simulink model "SimulinkMaster"  (R2025b)
settings: Solver=ode5  StartTime=0.0  StopTime=inf  RelTol=1e-3
undefined symbols (not defined in the file or in its folder): National_Instruments, PCI
libraries: sldrtlib x7, dspstat3 x3
settings Model: Creator=Admin  LastModifiedBy=Admin
settings HardwareCC: ProdBitPerLong=64.0  ProdHWDeviceType=Intel->x86-64 (Linux 64)
settings RTWCC: SystemTargetFile=sldrt.tlc  TemplateMakefile=sldrt.tmf  RTWCompilerOptimization=on  Description=Simulink Desktop Real-Time
settings CodeAppCC: MaxIdLength=95.0
settings SimulinkDesktopRealTimeCC: ExtModeTransport=0.0  ExtModeStaticAllocSize=1000000.0  TargetLibSuffix=_sldrt.a  TargetPreCompLibLocation=C:\Program Files\MATLAB\R2025b\toolbox\sldrt\lib\win64  MultiwordLength=2048.0  DynamicStringBufferSize=256.0  ParMdlRefBuildCompliant=on  PreserveMATLABNamespacesInGeneratedCode=on  SubcomponentCodeInterfacePackaging=Reusable function

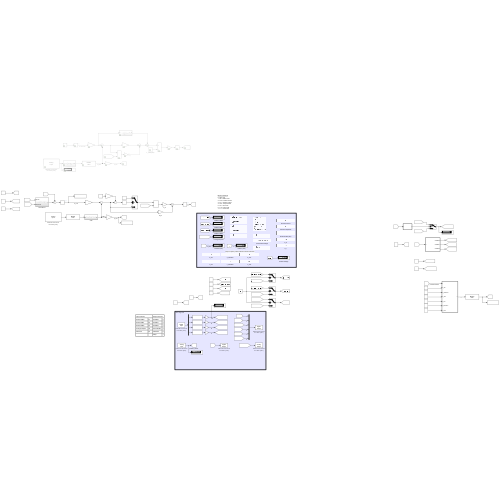
[thumbnail: Simulink's stored preview of the top-level diagram]
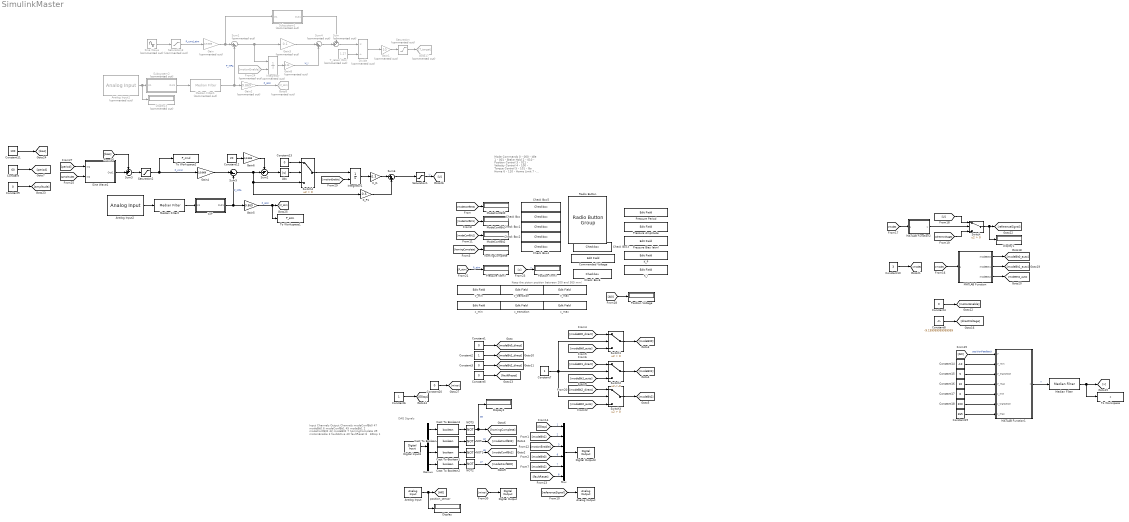
== system SimulinkMaster ==
  note: Keep the piston position between 200 and 365 mm!
  note: Input Channels
      | ​Output Channels
      |
      | modeConfBit0
      | 47
      | modeBit0
      | 6
      |
      | modeConfBit1
      | 45
      | modeBit1
      | 2
      |
      | modeConfBit2
      | 42
      | modeBit2
      | 7
      |
      | homingComplete
      | 39
      | motionEnable
      | 3
      |
      | faultActive
      | 40
      | faultReset
      | 8
      |
      | ​
      | ​
      | EStop
      | 1
  note: DAQ Signals
  note: Mode Commands
      | 0 - 000 - Idle
      | 1 - 001 - Brake Hold
      | 2 - 010 - Position Control
      | 3 - 011 - Velocity Control
      | 4 - 100 - Torque Control
      | 5 - 101 - Go Home
      | 6 - 110 - Home Limit
      | 7 - 111 - Home EOT
  Abs : Abs  SaturateOnIntegerOverflow=off
  Analog Input : sldrtlib/Analog Input  SampleTime=0.003  MaxMissedTicks=1e6  ShowMissedTicks=off  YieldWhenWaiting=off  DrvName=National_Instruments/PCI-6251  DrvAddress=4294967295  DrvOptions=[1 255 0 0 0]  Channels=[1]  RangeMode=1  VoltRange=1  DataType=1
      settings: AttributesFormatString=National Instruments\nPCI-6251 [auto]
  Analog Input1 : sldrtlib/Analog Input  Commented=on  SampleTime=0.003  MaxMissedTicks=1e6  ShowMissedTicks=off  YieldWhenWaiting=off  DrvName=National_Instruments/PCI-6251  DrvAddress=4294967295  DrvOptions=[1 255 0 0 0]  Channels=3  RangeMode=1  VoltRange=1  DataType=1
      settings: AttributesFormatString=National Instruments\nPCI-6251 [auto]
  Analog Input2 : sldrtlib/Analog Input  SampleTime=0.003  MaxMissedTicks=1e6  ShowMissedTicks=off  YieldWhenWaiting=off  DrvName=National_Instruments/PCI-6251  DrvAddress=4294967295  DrvOptions=[1 255 0 0 0]  Channels=3  RangeMode=1  VoltRange=1  DataType=1
      settings: AttributesFormatString=National Instruments\nPCI-6251 [auto]
  Analog Output : sldrtlib/Analog Output  SampleTime=0.003  MaxMissedTicks=1e6  ShowMissedTicks=off  YieldWhenWaiting=off  DrvName=National_Instruments/PCI-6251  DrvAddress=4294967295  DrvOptions=[1 255 0 0 0]  Channels=1  RangeMode=1  VoltRange=1  InitialValue=[]  FinalValue=[]
      settings: AttributesFormatString=National Instruments\nPCI-6251 [auto]
  Cast To Boolean{,1..3} (4 alike) : DataTypeConversion  OutDataTypeStr=boolean  SaturateOnIntegerOverflow=off  RndMeth=Floor
  Check Box : Checkbox  LabelPosition=Hide  ShowInitialText=on  Label=modeBit0  Values=[0.0, 1.0]
  Check Box1 : Checkbox  LabelPosition=Hide  ShowInitialText=on  Label=modeBit1  Values=[0.0, 1.0]
  Check Box2 : Checkbox  LabelPosition=Hide  ShowInitialText=on  Label=modeBit2  Values=[0.0, 1.0]
  Check Box3 : Checkbox  LabelPosition=Hide  ShowInitialText=on  Label=motionEnable  Values=[0.0, 1.0]
  Check Box4 : Checkbox  LabelPosition=Hide  ShowInitialText=on  Label=faultReset  Values=[0.0, 1.0]
  Check Box5 : Checkbox  LabelPosition=Hide  ShowInitialText=on  Label=Direct Control  Values=[0.0, 1.0]
  Check Box6 : Checkbox  LabelPosition=Hide  ShowInitialText=on  Label=Mixer  Values=[0.0, 1.0]
  Commanded Voltage : EditField  LabelPosition=Hide  ShowInitialText=on  Alignment=Center
  Constant : Constant  Value=60
  Constant{1,3..5,9,13,17,20} (8 alike) : Constant  Value=0
  Constant10 : Constant  Value=3
  Constant11 : Constant  Value=100
  Constant12 : Constant  Value=20
  Constant14 : Constant  Value=-10
  Constant15 : Constant  Value=5
  Constant16 : Constant  Value=10
  Constant18 : Constant  Value=200
  Constant19 : Constant  Value=365
  Constant2 : Constant
  Constant6 : Constant
  Constant7 : Constant
  Constant8 : Constant  Value=-9.199999999999999
  Demux : Demux
  Digital Input3 : sldrtlib/Digital Input  SampleTime=0.003  MaxMissedTicks=1e6  ShowMissedTicks=off  YieldWhenWaiting=off  DrvName=National_Instruments/PCI-6251  DrvAddress=4294967295  DrvOptions=[1 255 0 0 0]  Channels=[39,42,45,47]  BitMode=1  DataType=1
      settings: AttributesFormatString=National Instruments\nPCI-6251 [auto]
  Digital Output : sldrtlib/Digital Output  SampleTime=0.01  MaxMissedTicks=1e6  ShowMissedTicks=off  YieldWhenWaiting=off  DrvName=National_Instruments/PCI-6251  DrvAddress=4294967295  DrvOptions=[1 255 0 0 0]  Channels=5  BitMode=1  InitialValue=[]  FinalValue=[]
      settings: AttributesFormatString=National Instruments\nPCI-6251 [auto]
  Digital Output3 : sldrtlib/Digital Output  SampleTime=0.003  MaxMissedTicks=1e6  ShowMissedTicks=off  YieldWhenWaiting=off  DrvName=National_Instruments/PCI-6251  DrvAddress=4294967295  DrvOptions=[1 255 0 0 0]  Channels=[1,2,3,6,7,8]  BitMode=1  InitialValue=[0]  FinalValue=[0]
      settings: AttributesFormatString=National Instruments\nPCI-6251 [auto]
  Display : Display
  Display1 : Display
  Display2 : Display
  Display3 : Display  Commented=on
  Divide : Product  Commented=on  Inputs=*/
  From24 : From  Commented=on  GotoTag=motionEnable
  Gain : Gain  Commented=on  Gain=1/9.869
  Gain1 : Gain  Commented=on  Gain=10
  Gain2 : Gain  Commented=on  Gain=9.869
  Gain3 : Gain  Commented=on  Gain=0.1
  Gain4 : Gain  Gain=1/9.869
  Gain5 : Gain  Gain=9.869
  Gain6 : Gain  Gain=1/9.869
  Gain8 : Gain  Commented=on  Gain=0.05
  Goto17 : Goto  Commented=on  GotoTag=T_target
  Goto8 : Goto  Commented=on  GotoTag=P_atm
  Integrator : Integrator  Commented=on  ExternalReset=either  UpperSaturationLimit=1  LowerSaturationLimit=-1
  Integrator1 : Integrator  ExternalReset=either
  K_I : EditField  LabelPosition=Hide  ShowInitialText=on  Alignment=Center
  K_I1 : Gain  Gain=0.3
  K_P : EditField  LabelPosition=Hide  ShowInitialText=on  Alignment=Center
  K_P1 : Gain  Gain=0.5
  MATLAB Function : MATLAB Function  TreatAsAtomicUnit=on
  MATLAB Function1 : MATLAB Function  TreatAsAtomicUnit=on
  MATLAB Function2 : MATLAB Function  TreatAsAtomicUnit=on
  Median Filter : dspstat3/Median Filter  WindowLength=5  SimulateUsing=Interpreted execution
      settings: LibrarySourceBlock=|
      | dspfdesign/Median
      | Filter
  Median Filter1 : dspstat3/Median Filter  Commented=on  WindowLength=7  SimulateUsing=Interpreted execution
      settings: LibrarySourceBlock=|
      | dspfdesign/Median
      | Filter
  Median Filter2 : dspstat3/Median Filter  WindowLength=7  SimulateUsing=Interpreted execution
      settings: LibrarySourceBlock=|
      | dspfdesign/Median
      | Filter
  ModeConfBit0 : Display
  ModeConfBit1 : Display
  ModeConfBit2 : Display
  Mux : Mux  Inputs=6
  NOT{,1..3} (4 alike) : Logic  Operator=NOT  IconShape=distinctive  AllPortsSameDT=off  OutDataTypeStr=boolean
  Position (mm) : Display
  Position Voltage : Display
  Pressure (atm) : Display
  Pressure Amplitude : EditField  LabelPosition=Hide  ShowInitialText=on  Alignment=Center
  Pressure Bias (atm) : EditField  LabelPosition=Hide  ShowInitialText=on  Alignment=Center
  Pressure Period : EditField  LabelPosition=Hide  ShowInitialText=on  Alignment=Center
  Radio Button : RadioButtonGroup  LabelPosition=Hide  SelectedLabel=Velocity Control  ButtonGroupName=Mode Select
  Saturation : Saturate  Commented=on  UpperLimit=10  LowerLimit=-10
  Saturation1 : Saturate  UpperLimit=10  LowerLimit=-10
  Saturation2 : Saturate  UpperLimit=100  LowerLimit=5
  Saturation3 : Saturate  Commented=on  UpperLimit=100  LowerLimit=5
  Sine Wave : Sin  Commented=on  Amplitude=15  Bias=60  Frequency=2*pi*0.025  SampleTime=0
  Sine Wave1 : Subsystem
  Subsystem1 : Subsystem  Commented=on
  Subsystem2 : Subsystem  Commented=on
  Sum : Sum  Commented=on  Inputs=++|
  Sum1 : Sum  Commented=on  Inputs=|+-
  Sum2 : Sum  Inputs=-+|
  Sum3 : Sum  Inputs=++|
  Sum4 : Sum  Commented=on  Inputs=|++
  Sum5 : Sum  Inputs=|+-
  Sum6 : Sum  Inputs=|++
  Switch{,1..4} (5 alike) : Switch  Criteria=u2 > Threshold  SaturateOnIntegerOverflow=off  InputSameDT=off
  T_rated (Nm) : Constant  Commented=on  Value=1.27
  To Workspace : ToWorkspace  VariableName=x  SaveFormat=Timeseries  SampleTime=-1
  To Workspace1 : ToWorkspace  VariableName=P_atm  SaveFormat=Timeseries  SampleTime=-1
  To Workspace2 : ToWorkspace  VariableName=P_cmd  SaveFormat=Timeseries  SampleTime=-1
  V2P : Subsystem
  V_max : EditField  LabelPosition=Hide  ShowInitialText=on  Alignment=Center
  V_min : EditField  LabelPosition=Hide  ShowInitialText=on  Alignment=Center
  V_transition : EditField  LabelPosition=Hide  ShowInitialText=on  Alignment=Center
  homingComplete : Display
  x_max : EditField  LabelPosition=Hide  ShowInitialText=on  Alignment=Center
  x_min : EditField  LabelPosition=Hide  ShowInitialText=on  Alignment=Center
  x_transition : EditField  LabelPosition=Hide  ShowInitialText=on  Alignment=Center
  wires:
  Digital Input3/1 -> Demux/1
  Demux/2 -> Cast To Boolean/1
  Demux/3 -> Cast To Boolean1/1
  Demux/4 -> Cast To Boolean2/1
  [modeBit1] -> Mux/2  "2"
  Mux/1 -> Digital Output3/1
  [modeConfBit0] -> ModeConfBit0/1
  [modeConfBit1] -> ModeConfBit1/1
  [modeConfBit2] -> ModeConfBit2/1
  Constant1/1 -> [modeBit0_direct]
  Constant2/1 -> [modeBit1_direct]
  Constant3/1 -> [modeBit2_direct]
  NOT/1 -> [modeConfBit2]  "42"
  NOT1/1 -> [modeConfBit1]  "45"
  NOT2/1 -> [modeConfBit0]  "47"
  Cast To Boolean/1 -> NOT/1
  Cast To Boolean1/1 -> NOT1/1
  Cast To Boolean2/1 -> NOT2/1
  [modeBit2] -> Mux/5  "7"
  [modeBit0] -> Mux/4  "6"
  Constant4/1 -> [motionEnable]
  [motionEnable] -> Mux/3  "3"
  [faultReset] -> Mux/6  "8"
  Constant5/1 -> [faultReset]
  Constant6/1 -> [EStop]
  [EStop] -> Mux/1  "1"
  Demux/1 -> Cast To Boolean3/1
  Cast To Boolean3/1 -> NOT3/1
  NOT3/1 -> Display2/1, [homingComplete]  "39"
  [homingComplete] -> homingComplete/1
  [referenceSignal] -> Analog Output/1
  MATLAB Function/3(modeBit2) -> [modeBit2_auto]
  MATLAB Function/2(modeBit1) -> [modeBit1_auto]
  MATLAB Function/1(modeBit0) -> [modeBit0_auto]
  [AI0] -> MATLAB Function1/1(V)  "positionFeedback"
  MATLAB Function1/1(x) -> Median Filter/1  "x"
  Analog Input/1 -> Display/1, [AI0]
  Constant8/1 -> [directVoltage]
  Gain1/1 -> Saturation/1
  Saturation/1 -> Goto17/1
  Divide/1 -> Gain1/1
  T_rated (Nm)/1 -> Divide/2
  Subsystem2/1(Out1) -> Median Filter1/1
  Analog Input1/1 -> Display3/1, Subsystem2/1(In1)
  Subsystem1/1(Out1) -> Sum/1
  Gain/1 -> Sum1/1, Subsystem1/1(In1)
  Constant10/1 -> [mode]
  [mode] -> MATLAB Function/1(u)
  [mode] -> MATLAB Function2/1(u)
  MATLAB Function2/1(y) -> Switch/2
  [directVoltage] -> Switch/3
  [U] -> Switch/1
  Switch/1 -> [referenceSignal], Display1/1
  [modeBit0_direct] -> Switch1/1
  [modeBit0_auto] -> Switch1/3
  [modeBit1_direct] -> Switch2/1
  [modeBit1_auto] -> Switch2/3
  [modeBit2_direct] -> Switch3/1
  [modeBit2_auto] -> Switch3/3
  Switch1/1 -> [modeBit0]
  Switch2/1 -> [modeBit1]
  Switch3/1 -> [modeBit2]
  Constant7/1 -> Switch3/2, Switch1/2, Switch2/2
  Gain2/1 -> Goto8/1  "P_atm"
  Median Filter1/1 -> Gain2/1, Sum1/2  "P_MPa"
  Sum1/1 -> Gain3/1, Integrator/1
  Integrator/1 -> Gain8/1
  Gain3/1 -> Sum4/1
  Gain8/1 -> Sum4/2  "U_I"
  Sum4/1 -> Sum/2
  [P_atm] -> Pressure (atm)/1  "P_atm"
  [x] -> Position (mm)/1  "x"
  Saturation3/1 -> Gain/1  "P_cmd_atm"
  From24/1 -> Integrator/2
  Sum/1 -> Divide/1
  Median Filter/1 -> To Workspace/1, [x]
  Sine Wave/1 -> Saturation3/1
  Sum6/1 -> Saturation1/1
  Saturation2/1 -> To Workspace2/1, Gain4/1  "P_cmd"
  Saturation1/1 -> [U]  "U"
  [motionEnable] -> Integrator1/2
  K_P1/1 -> Sum6/2
  K_I1/1 -> Sum6/1
  Switch4/1 -> Integrator1/1
  Gain6/1 -> Sum2/1
  Sum5/1 -> Sum2/2, K_P1/1, Switch4/3
  Constant13/1 -> Switch4/1
  Abs/1 -> Switch4/2
  Sum2/1 -> Abs/1
  Constant12/1 -> Gain6/1
  Gain4/1 -> Sum5/1
  Sum3/1 -> Saturation2/1
  Gain5/1 -> To Workspace1/1, [P_atm]  "P_atm"
  V2P/1(Out1) -> Gain5/1, Sum5/2  "P_MPa"
  Median Filter2/1 -> V2P/1(In1)
  Analog Input2/1 -> Median Filter2/1
  Constant11/1 -> [bias]
  [amplitude] -> Sine Wave1/2(In2)
  [period] -> Sine Wave1/1(In1)
  [bias] -> Sum3/1
  Sine Wave1/1(Out1) -> Sum3/2
  Constant9/1 -> [amplitude]
  Constant/1 -> [period]
  Integrator1/1 -> K_I1/1
  Constant14/1 -> MATLAB Function1/2(V_min)
  Constant15/1 -> MATLAB Function1/3(V_transition)
  Constant16/1 -> MATLAB Function1/4(V_max)
  Constant17/1 -> MATLAB Function1/5(x_min)
  Constant18/1 -> MATLAB Function1/6(x_transition)
  Constant19/1 -> MATLAB Function1/7(x_max)
  [AI0] -> Position Voltage/1
  [mixer] -> Digital Output/1
  Constant20/1 -> [mixer]

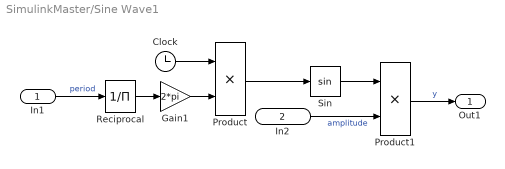
== system SimulinkMaster/Sine Wave1 ==
  In1 : Inport
  In2 : Inport  Port=2
  Clock : Clock
  Gain1 : Gain  Gain=2*pi
  Product : Product
  Product1 : Product
  Reciprocal : Product  Inputs=/
  Sin : Trigonometry
  Out1 : Outport
  wires:
  Clock/1 -> Product/1
  In2/1 -> Product1/2  "amplitude"
  Gain1/1 -> Product/2
  Product1/1 -> Out1/1  "y"
  Product/1 -> Sin/1
  Reciprocal/1 -> Gain1/1
  In1/1 -> Reciprocal/1  "period"
  Sin/1 -> Product1/1

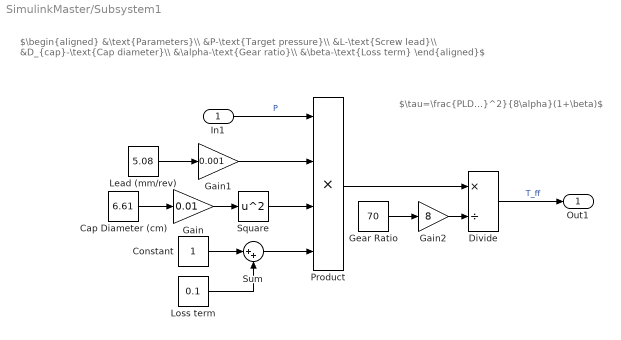
== system SimulinkMaster/Subsystem1 ==
  note: $\tau=\frac{PLD_{cap}^2}{8\alpha}(1+\beta)$
  note: $\begin{aligned} &\text{Parameters}\\ &P-\text{Target pressure}\\ &L-\text{Screw lead}\\ &D_{cap}-\text{Cap diameter}\\ &\alpha-\text{Gear ratio}\\ &\beta-\text{Loss term} \end{aligned}$
  In1 : Inport
  Cap Diameter (cm) : Constant  Value=6.61
  Constant : Constant
  Divide : Product  Inputs=*/
  Gain : Gain  Gain=0.01
  Gain1 : Gain  Gain=0.001
  Gain2 : Gain  Gain=8
  Gear Ratio : Constant  Value=70
  Lead (mm/rev) : Constant  Value=5.08
  Loss term : Constant  Value=0.1
  Product : Product  Inputs=4
  Square : Math  Operator=square
  Sum : Sum  Inputs=|++
  Out1 : Outport
  wires:
  Gain2/1 -> Divide/2
  Gear Ratio/1 -> Gain2/1
  Divide/1 -> Out1/1  "T_ff"
  Product/1 -> Divide/1
  Gain1/1 -> Product/2
  Lead (mm/rev)/1 -> Gain1/1
  In1/1 -> Product/1  "P"
  Square/1 -> Product/3
  Sum/1 -> Product/4
  Gain/1 -> Square/1
  Cap Diameter (cm)/1 -> Gain/1
  Loss term/1 -> Sum/2
  Constant/1 -> Sum/1

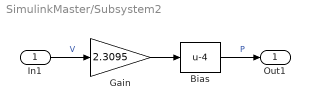
== system SimulinkMaster/Subsystem2 ==
  In1 : Inport
  Bias : Bias  Bias=-4  SaturateOnIntegerOverflow=off
  Gain : Gain  Gain=2.3095
  Out1 : Outport
  wires:
  In1/1 -> Gain/1  "V"
  Gain/1 -> Bias/1
  Bias/1 -> Out1/1  "P"

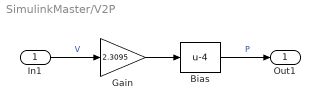
== system SimulinkMaster/V2P ==
  In1 : Inport
  Bias : Bias  Bias=-4  SaturateOnIntegerOverflow=off
  Gain : Gain  Gain=2.3095
  Out1 : Outport
  wires:
  In1/1 -> Gain/1  "V"
  Bias/1 -> Out1/1  "P"
  Gain/1 -> Bias/1

== matlab function SimulinkMaster/MATLAB Function ==
  data: u input; modeBit0 output; modeBit1 output; modeBit2 output
function [modeBit0,modeBit1,modeBit2] = fcn(u)

if u == 0
    modeBit2 = 0;
    modeBit1 = 0;
    modeBit0 = 0;
elseif u == 6
    modeBit2 = 1;
    modeBit1 = 1;
    modeBit0 = 0;
elseif u == 2
    modeBit2 = 0;
    modeBit1 = 1;
    modeBit0 = 0;
elseif u == 3
    modeBit2 = 0;
    modeBit1 = 1;
    modeBit0 = 1;
elseif u == 4
    % modeBit2 = 1; Torque control
    % modeBit1 = 0;
    % modeBit0 = 0;
    modeBit2 = 0; % Use velocity control instead
    modeBit1 = 1;
    modeBit0 = 1;
else
    modeBit2 = 0;
    modeBit1 = 0;
    modeBit0 = 0;
end

== matlab function SimulinkMaster/MATLAB Function2 ==
  data: u input; y output
function y = fcn(u)

if u == 4
    y = 1;
else
    y = 0;
end

== matlab function SimulinkMaster/MATLAB Function1 ==
  data: V input; x output; V_min input; V_transition input; V_max input; x_min input; x_transition input; x_max input
function x = V2x(V,V_min,V_transition,V_max,x_min,x_transition,x_max)

if V <= V_transition
    x = (V-V_min)*(x_transition-x_min)/(V_transition-V_min)+x_min;
else
    x = (V-V_transition)*(x_max-x_transition)/(V_max-V_transition)+x_transition;
end
